simulink model "Reference_model_Control_Engineering_Feedforward"  (R2019b)
settings: Solver=FixedStepDiscrete  StartTime=0.0  StopTime=inf  FixedStep=Ts  RelTol=1e-3  EnableMultiTasking=on
InitFcn:
  | Fs = 4000; Ts = 1/Fs; tsim = 29.9997;
libraries: sperte_lib x3
settings Model: SimulationMode=external  Creator=Enzo  LastModifiedBy=20182597
settings SolverCC: PositivePriorityOrder=on
settings DataIOCC: SaveOutput=off  DSMLogging=off  SaveTime=off  ReturnWorkspaceOutputs=off
settings OptimizationCC: EnhancedBackFolding=on  PassReuseOutputArgsThreshold=0  MaxStackSize=64  OptimizeBlockOrder=speed  DifferentSizesBufferReuse=on  OptimizationCustomize=off
settings DebuggingCC: ParameterTunabilityLossMsg=error  ArithmeticOperatorsInVariantConditions=warning
settings HardwareCC: ProdBitPerPointer=32  ProdBitPerSizeT=32  ProdBitPerPtrDiffT=32  ProdLargestAtomicInteger=Long  ProdLargestAtomicFloat=Double  ProdWordSize=32  ProdLongLongMode=on  ProdHWDeviceType=ARM Compatible->ARM Cortex  UseEmbeddedCoderFeatures=off
settings SFSimCC: CustomCodeUndefinedFunction=UseInterfaceOnly
settings RTWCC: SystemTargetFile=ert.tlc  HardwareBoard=Raspberry Pi  TLCOptions="-aInlineSetEventsForThisBaseRateFcn=TLC_FALSE -aSuppressMultiTaskScheduler=TLC_FALSE  -aRateBasedStepFcn=0"  TemplateMakefile=ert_default_tmf  PostCodeGenCommand="if (~verLessThan('matlab', '9.11')) codertarget.postCodeGenHookCommand(h);  SPERTE_postGenFunc(modelName, buildInfo); else; SPERTE_postGenFunc(h, buildInfo); end"  Toolchain=GNU GCC Raspberry Pi  BuildConfiguration=Faster Runs
settings CodeAppCC: ForceParamTrailComments=on  OperatorAnnotations=on
settings ERTTargetCC: ERTCustomFileBanners=off  SupportContinuousTime=on  SupportNonInlinedSFcns=on  RemoveResetFunc=off  SupportVariableSizeSignals=on  ModelStepFunctionPrototypeControlCompliant=off  ExtMode=on  ExtModeMexArgs='sperte0.bwk.tue.nl' 0 17725  ERTSrcFileBannerTemplate=codertarget_code_template.cgt  ERTHdrFileBannerTemplate=codertarget_code_template.cgt  ERTDataSrcFileTemplate=codertarget_code_template.cgt  ERTDataHdrFileTemplate=codertarget_code_template.cgt

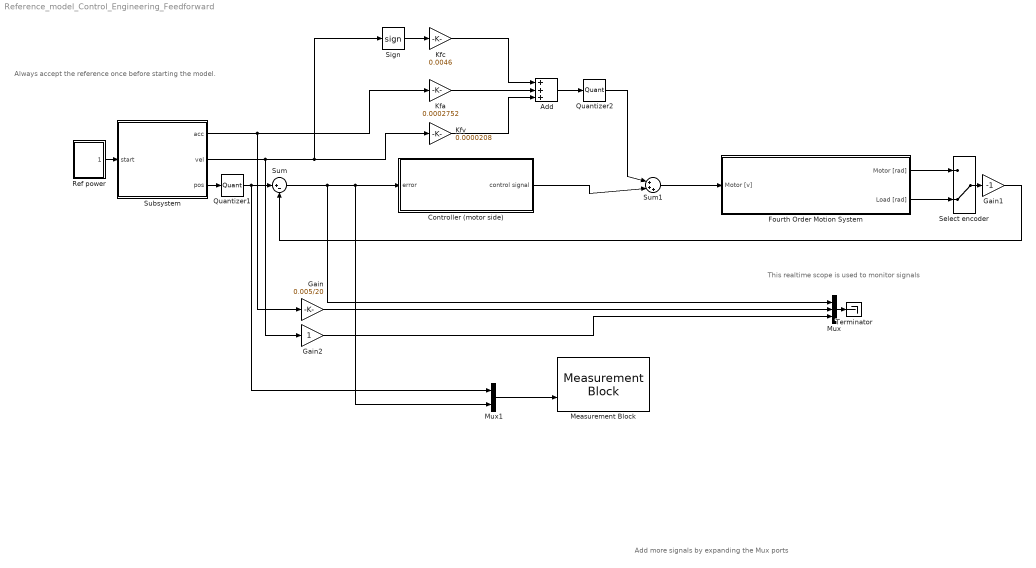
== system Reference_model_Control_Engineering_Feedforward ==
  note: Add more signals by expanding the Mux ports
  note: This realtime scope is used to monitor signals
  note: Always accept the reference once before starting the model.
  Add : Sum  Inputs=+++
  Controller (motor side) : Subsystem
  Fourth Order Motion System : Subsystem
  Gain : Gain  Gain=0.005/20
  Gain1 : Gain  Gain=-1
  Gain2 : Gain
  Kfa : Gain  Gain=0.0002752
  Kfc : Gain  Gain=0.0046
  Kfv : Gain  Gain=0.0000208
  Measurement Block : sperte_lib/Measurement Block  Description=|  Priority=-1  N_samples=500000  triggertype=2  trigger_command=0
      | Perform on-demand measurements to file using this block.
      | 
      | It can be used in 2 ways:
      | 1) Set the mask triggertype parameter to manual and use the trigger input signal to trigger a measurement.
      | You can do this by providing a 0 to 1 transition.
      | Keep it low after you start/complete the measurement, or it will measure again.
      | A file is created with measurement_0,1,2... etc
      | 
      | 2) Keep the model running, and trigger a measurement from the commandline or Matlab script.
      | For example:
      | 
      | % How many samples to measure?
      | N_samples = Fs*5;
      | % Do the measurement
      | SPERTE_Perform_Measurement(N_samples);
      | % Get the latest file
      | file_list = SPERTE_Get_Latest_Measurement(p,1,'./data');
      | % How many signals did you record?
      | N_signals = 3;
      | % Convert the .bin to .mat and return the results
      | measurement = SPERTE_Bin_To_Mat(file_list,N_signals);
      settings: SourceProductName=SPERTE project library
  Mux : Mux  Inputs=3
  Mux1 : Mux  Inputs=2
  Quantizer1 : Quantizer  QuantizationInterval=(2*pi)/(500*4)
  Quantizer2 : Quantizer  QuantizationInterval=(2*pi)/(500*4)
  Ref power : Subsystem  mask(On/Off Switch){stat=On}
      mask prompts: stat "Switch"
      mask TypeOptions stat: On | Off
  Select encoder : ManualSwitch  CurrentSetting=0
  Sign : Signum
  Subsystem : Subsystem  mask(Ref3){}
      settings: OpenFcn=global ref_part; cb_axes 1
      mask Display: disp('Ref3');
  Sum : Sum  Inputs=|+-
  Sum1 : Sum  Inputs=|+++
  Terminator : Terminator
  wires:
  Fourth Order Motion System/1(Motor [rad]) -> Select encoder/1
  Fourth Order Motion System/2(Load [rad]) -> Select encoder/2
  Sum1/1 -> Fourth Order Motion System/1(Motor [v])
  Sum/1 -> Mux/1, Mux1/2, Controller (motor side)/1(error)
  Quantizer1/1 -> Mux1/1, Sum/1
  Ref power/1(On/Off) -> Subsystem/1(start)
  Subsystem/3(pos) -> Quantizer1/1
  Kfc/1 -> Add/1
  Kfa/1 -> Add/2
  Kfv/1 -> Add/3
  Controller (motor side)/1(control signal) -> Sum1/2
  Add/1 -> Quantizer2/1
  Quantizer2/1 -> Sum1/1
  Subsystem/1(acc) -> Kfa/1, Gain/1
  Subsystem/2(vel) -> Sign/1, Kfv/1, Gain2/1
  Sign/1 -> Kfc/1
  Mux/1 -> Terminator/1
  Gain/1 -> Mux/2
  Select encoder/1 -> Gain1/1
  Gain1/1 -> Sum/2
  Mux1/1 -> Measurement Block/2
  Gain2/1 -> Mux/3

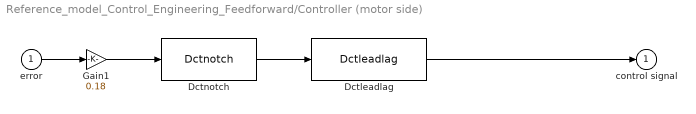
== system Reference_model_Control_Engineering_Feedforward/Controller (motor side) ==
  error : Inport
  Dctleadlag : sperte_lib/Dctleadlag  f_num=1  f_den=100
      settings: SourceProductName=SPERTE project library
  Dctnotch : sperte_lib/Dctnotch  f_num=59  b_num=0.005  f_den=59  b_den=.5
      settings: SourceProductName=SPERTE project library
  Gain1 : Gain  Gain=0.18  SaturateOnIntegerOverflow=on  OutDataTypeStr=Inherit: Same as input  ParamDataTypeStr=Inherit: Same as input
  control signal : Outport
  wires:
  Dctleadlag/1 -> control signal/1
  Gain1/1 -> Dctnotch/1
  error/1 -> Gain1/1
  Dctnotch/1 -> Dctleadlag/1

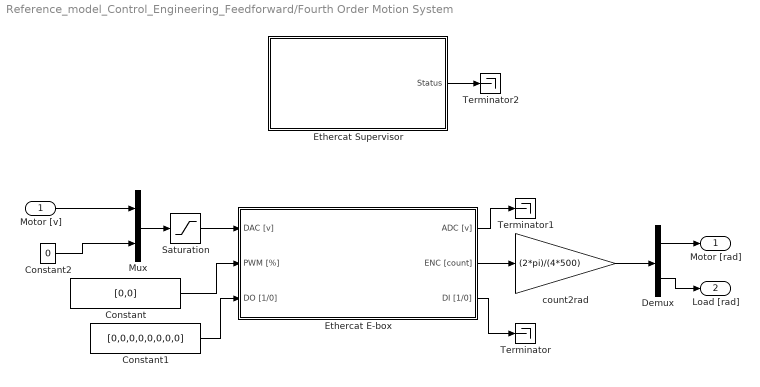
== system Reference_model_Control_Engineering_Feedforward/Fourth Order Motion System ==
  Motor [v] : Inport
  Constant : Constant  Value=[0,0]
  Constant1 : Constant  Value=[0,0,0,0,0,0,0,0]
  Constant2 : Constant  Value=0
  Demux : Demux  Outputs=2
  Ethercat E-box : Subsystem  Priority=-2  mask(Sperte Lib){link_id=0}
      mask prompts: link_id "Link ID of the specific ebox"
      mask help:
      | This block implements a single E-box device.
      | Ensure that if you have multiple E-box devices that they each have an unique link_id.
      |
      | You MUST have an Ethercat Initialize block in your model to be able to use this block.
      mask Display: ud = get_param(gcb,'UserData');image(ud.x);
  Ethercat Supervisor : Subsystem  Description=Must be executed first, keep at -1 priority (highest)  Priority=-3  mask(Sperte Lib){portid=0, ectimeout=500}
      mask prompts: portid "Ethernet port number for the Ethercat protocol (default 0 = eth0)"; ectimeout "Timeout of the Ethercat protocol in microseconds."
      mask help:
      | This block initializes the Ethercat connection on the Raspberry Pi.
      |
      | This enables you to use multiple E-box devices by including multiple blocks of the "Ethercat E-box" type.
      mask Display: ud = get_param(gcb,'UserData');image(ud.x);
  Mux : Mux  Inputs=2
  Saturation : Saturate  UpperLimit=2.5  LowerLimit=-2.5
  Terminator : Terminator
  Terminator1 : Terminator
  Terminator2 : Terminator
  count2rad : Gain  Gain=(2*pi)/(4*500)
  Motor [rad] : Outport
  Load [rad] : Outport  Port=2
  wires:
  Ethercat E-box/1(ADC [v]) -> Terminator1/1
  Ethercat E-box/2(ENC [count]) -> count2rad/1
  Constant/1 -> Ethercat E-box/2(PWM [%])
  Mux/1 -> Saturation/1
  count2rad/1 -> Demux/1
  Motor [v]/1 -> Mux/1
  Constant2/1 -> Mux/2
  Demux/1 -> Motor [rad]/1
  Demux/2 -> Load [rad]/1
  Ethercat E-box/3(DI [1/0]) -> Terminator/1
  Constant1/1 -> Ethercat E-box/3(DO [1/0])
  Saturation/1 -> Ethercat E-box/1(DAC [v])
  Ethercat Supervisor/1(Status) -> Terminator2/1

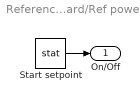
== system Reference_model_Control_Engineering_Feedforward/Ref power ==
  Start setpoint : Constant  Value=stat
  On/Off : Outport
  wires:
  Start setpoint/1 -> On/Off/1

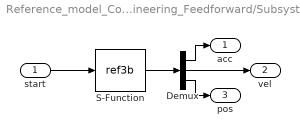
== system Reference_model_Control_Engineering_Feedforward/Subsystem ==
  start : Inport
  Demux : Demux  Outputs=3
  S-Function : S-Function  FunctionName=ref3b  Parameters=ref_part  SFunctionDeploymentMode=off  EnableBusSupport=off
      settings: OpenFcn=global ref_part; r3g_main
  acc : Outport
  vel : Outport  Port=2
  pos : Outport  Port=3
  wires:
  S-Function/1 -> Demux/1
  Demux/1 -> acc/1
  Demux/2 -> vel/1
  Demux/3 -> pos/1
  start/1 -> S-Function/1

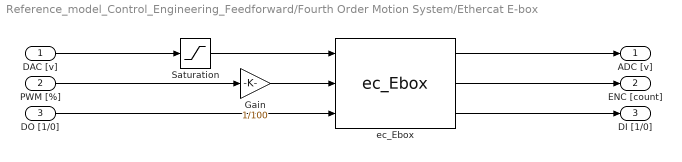
== system Reference_model_Control_Engineering_Feedforward/Fourth Order Motion System/Ethercat E-box ==
  DAC [v] : Inport
  PWM [%] : Inport  Port=2
  DO [1/0] : Inport  Port=3
  Gain : Gain  Gain=1/100
  Saturation : Saturate  UpperLimit=10  LowerLimit=-10
  ec_Ebox : S-Function  FunctionName=ec_Ebox  Parameters=link_id  SFunctionDeploymentMode=off  EnableBusSupport=off  mask{link_id=link_id}
      mask prompts: link_id "link_id >= 0"
      mask Display:
      | port_label('output',1,'ADC')
      | port_label('output',2,'ENC')
      | port_label('output',3,'DI')
      | port_label('input',1,'DAC')
      | port_label('input',2,'PWM')
      | port_label('input',3,'DO')
  ADC [v] : Outport
  ENC [count] : Outport  Port=2
  DI [1/0] : Outport  Port=3
  wires:
  Gain/1 -> ec_Ebox/2
  Saturation/1 -> ec_Ebox/1
  ec_Ebox/3 -> DI [1/0]/1
  ec_Ebox/1 -> ADC [v]/1
  ec_Ebox/2 -> ENC [count]/1
  DAC [v]/1 -> Saturation/1
  DO [1/0]/1 -> ec_Ebox/3
  PWM [%]/1 -> Gain/1

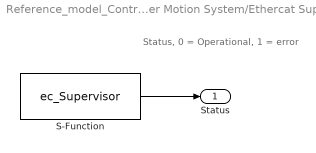
== system Reference_model_Control_Engineering_Feedforward/Fourth Order Motion System/Ethercat Supervisor ==
  note: Status, 0 = Operational, 1 = error
  S-Function : S-Function  FunctionName=ec_Supervisor  Parameters=portid,ectimeout  SFunctionDeploymentMode=off  EnableBusSupport=off
  Status : Outport
  wires:
  S-Function/1 -> Status/1
